simulink model "EHB_speedgoat_R2020a_V1"  (R2020a)
settings: Solver=FixedStepDiscrete  StartTime=0.0  StopTime=inf  FixedStep=0.001  RelTol=1e-3  EnableMultiTasking=on
model workspace (MAT data in the model file):
  A : Simulink.Signal (value not decoded)
  B : Simulink.Signal (value not decoded)
  C : Simulink.Signal (value not decoded)
  D : Simulink.Signal (value not decoded)
  E : Simulink.Signal (value not decoded)
  calin = [-9.96 -7.98 -5.98 -3.99 -1.994 0 1.995 3.992 5.99 7.98 9.97]
  calout = [-10 -8 -6 -4 -2 0 2 4 6 8 10]
symbols that are objects in the model workspace (value not decoded): C, D
undefined symbols (not defined in the file): Com1, none, ts_IO612
libraries: simulink x1436, xpcethercatlib x1223, yisutbxlib_utilities x256, xpcutilitieslib x156, hdlsllib x145, canmsglib x46, speedgoatlib_IO602_4 x11, speedgoatlib_IO611 x7, slrttcplib x4, CanManageLib x3, slrtlib x3, xpcseriallib x2
(part 4 of 30)

== system EHB_speedgoat_R2020a_V1/TIF_04/CB2020_2/mean11 ==
  In1 : Inport
  Add : Sum  Inputs=++++
  Add{1..4} (4 alike) : Sum  Inputs=++++++++++++++++++++
  Delay{,1..79} (80 alike) : Delay  DelayLength=1
  Gain : Gain  Gain=1/80
  Vol : Outport
  wires:
  Add/1 -> Gain/1
  Gain/1 -> Vol/1
  Delay36/1 -> Delay37/1, Add2/7
  Delay37/1 -> Delay38/1, Add2/8
  Delay34/1 -> Delay35/1, Add2/5
  Delay33/1 -> Delay34/1, Add2/4
  Delay20/1 -> Delay21/1, Add2/1
  Delay32/1 -> Delay33/1, Add2/3
  Add2/1 -> Add/2
  Delay35/1 -> Delay36/1, Add2/6
  Delay21/1 -> Delay32/1, Add2/2
  Delay38/1 -> Delay39/1, Add2/9
  Delay39/1 -> Delay22/1, Add2/10
  Delay19/1 -> Add1/20, Delay20/1
  Delay30/1 -> Delay31/1, Add2/19
  Delay23/1 -> Delay24/1, Add2/12
  Delay27/1 -> Delay28/1, Add2/16
  Delay24/1 -> Delay25/1, Add2/13
  Delay22/1 -> Delay23/1, Add2/11
  Delay25/1 -> Delay26/1, Add2/14
  Delay26/1 -> Delay27/1, Add2/15
  Delay29/1 -> Delay30/1, Add2/18
  Delay28/1 -> Delay29/1, Add2/17
  Delay16/1 -> Add1/17, Delay17/1
  Delay17/1 -> Add1/18, Delay18/1
  Delay14/1 -> Add1/15, Delay15/1
  Delay13/1 -> Add1/14, Delay14/1
  Delay10/1 -> Add1/11, Delay11/1
  Delay12/1 -> Add1/13, Delay13/1
  Delay15/1 -> Add1/16, Delay16/1
  Delay11/1 -> Add1/12, Delay12/1
  Delay18/1 -> Add1/19, Delay19/1
  In1/1 -> Delay/1
  Delay9/1 -> Add1/10, Delay10/1
  Delay8/1 -> Add1/9, Delay9/1
  Delay1/1 -> Add1/2, Delay2/1
  Delay5/1 -> Add1/6, Delay6/1
  Add1/1 -> Add/1
  Delay2/1 -> Add1/3, Delay3/1
  Delay/1 -> Add1/1, Delay1/1
  Delay3/1 -> Add1/4, Delay4/1
  Delay4/1 -> Add1/5, Delay5/1
  Delay7/1 -> Add1/8, Delay8/1
  Delay6/1 -> Add1/7, Delay7/1
  Delay48/1 -> Add3/17, Delay49/1
  Delay49/1 -> Add3/18, Delay50/1
  Delay46/1 -> Add3/15, Delay47/1
  Delay45/1 -> Add3/14, Delay46/1
  Delay42/1 -> Add3/11, Delay43/1
  Delay44/1 -> Add3/13, Delay45/1
  Delay47/1 -> Add3/16, Delay48/1
  Delay43/1 -> Add3/12, Delay44/1
  Delay50/1 -> Add3/19, Delay51/1
  Delay31/1 -> Delay40/1, Add2/20
  Delay59/1 -> Add3/10, Delay42/1
  Delay58/1 -> Add3/9, Delay59/1
  Delay41/1 -> Add3/2, Delay52/1
  Delay55/1 -> Add3/6, Delay56/1
  Add3/1 -> Add/3
  Delay52/1 -> Add3/3, Delay53/1
  Delay40/1 -> Add3/1, Delay41/1
  Delay53/1 -> Add3/4, Delay54/1
  Delay54/1 -> Add3/5, Delay55/1
  Delay57/1 -> Add3/8, Delay58/1
  Delay56/1 -> Add3/7, Delay57/1
  Delay76/1 -> Delay77/1, Add4/7
  Delay77/1 -> Delay78/1, Add4/8
  Delay74/1 -> Delay75/1, Add4/5
  Delay73/1 -> Delay74/1, Add4/4
  Delay60/1 -> Delay61/1, Add4/1
  Delay72/1 -> Delay73/1, Add4/3
  Add4/1 -> Add/4
  Delay75/1 -> Delay76/1, Add4/6
  Delay61/1 -> Delay72/1, Add4/2
  Delay78/1 -> Delay79/1, Add4/9
  Delay79/1 -> Delay62/1, Add4/10
  Delay71/1 -> Add4/20
  Delay51/1 -> Delay60/1, Add3/20
  Delay70/1 -> Delay71/1, Add4/19
  Delay63/1 -> Delay64/1, Add4/12
  Delay67/1 -> Delay68/1, Add4/16
  Delay64/1 -> Delay65/1, Add4/13
  Delay62/1 -> Delay63/1, Add4/11
  Delay65/1 -> Delay66/1, Add4/14
  Delay66/1 -> Delay67/1, Add4/15
  Delay69/1 -> Delay70/1, Add4/18
  Delay68/1 -> Delay69/1, Add4/17

== system EHB_speedgoat_R2020a_V1/TIF_04/CB2020_2/mean12 ==
  In1 : Inport
  Add : Sum  Inputs=++++
  Add{1..4} (4 alike) : Sum  Inputs=++++++++++++++++++++
  Delay{,1..79} (80 alike) : Delay  DelayLength=1
  Gain : Gain  Gain=1/80
  Vol : Outport
  wires:
  Delay68/1 -> Add4/17, Delay69/1
  Delay69/1 -> Add4/18, Delay70/1
  Delay66/1 -> Add4/15, Delay67/1
  Delay65/1 -> Add4/14, Delay66/1
  Delay62/1 -> Add4/11, Delay63/1
  Delay64/1 -> Add4/13, Delay65/1
  Delay67/1 -> Add4/16, Delay68/1
  Delay63/1 -> Add4/12, Delay64/1
  Delay70/1 -> Add4/19, Delay71/1
  Delay51/1 -> Add3/20, Delay60/1
  Delay71/1 -> Add4/20
  Delay79/1 -> Add4/10, Delay62/1
  Delay78/1 -> Add4/9, Delay79/1
  Delay61/1 -> Add4/2, Delay72/1
  Delay75/1 -> Add4/6, Delay76/1
  Add4/1 -> Add/4
  Delay72/1 -> Add4/3, Delay73/1
  Delay60/1 -> Add4/1, Delay61/1
  Delay73/1 -> Add4/4, Delay74/1
  Delay74/1 -> Add4/5, Delay75/1
  Delay77/1 -> Add4/8, Delay78/1
  Delay76/1 -> Add4/7, Delay77/1
  Delay56/1 -> Delay57/1, Add3/7
  Delay57/1 -> Delay58/1, Add3/8
  Delay54/1 -> Delay55/1, Add3/5
  Delay53/1 -> Delay54/1, Add3/4
  Delay40/1 -> Delay41/1, Add3/1
  Delay52/1 -> Delay53/1, Add3/3
  Add3/1 -> Add/3
  Delay55/1 -> Delay56/1, Add3/6
  Delay41/1 -> Delay52/1, Add3/2
  Delay58/1 -> Delay59/1, Add3/9
  Delay59/1 -> Delay42/1, Add3/10
  Delay31/1 -> Add2/20, Delay40/1
  Delay50/1 -> Delay51/1, Add3/19
  Delay43/1 -> Delay44/1, Add3/12
  Delay47/1 -> Delay48/1, Add3/16
  Delay44/1 -> Delay45/1, Add3/13
  Delay42/1 -> Delay43/1, Add3/11
  Delay45/1 -> Delay46/1, Add3/14
  Delay46/1 -> Delay47/1, Add3/15
  Delay49/1 -> Delay50/1, Add3/18
  Delay48/1 -> Delay49/1, Add3/17
  Delay6/1 -> Delay7/1, Add1/7
  Delay7/1 -> Delay8/1, Add1/8
  Delay4/1 -> Delay5/1, Add1/5
  Delay3/1 -> Delay4/1, Add1/4
  Delay/1 -> Delay1/1, Add1/1
  Delay2/1 -> Delay3/1, Add1/3
  Add1/1 -> Add/1
  Delay5/1 -> Delay6/1, Add1/6
  Delay1/1 -> Delay2/1, Add1/2
  Delay8/1 -> Delay9/1, Add1/9
  Delay9/1 -> Delay10/1, Add1/10
  In1/1 -> Delay/1
  Delay18/1 -> Delay19/1, Add1/19
  Delay11/1 -> Delay12/1, Add1/12
  Delay15/1 -> Delay16/1, Add1/16
  Delay12/1 -> Delay13/1, Add1/13
  Delay10/1 -> Delay11/1, Add1/11
  Delay13/1 -> Delay14/1, Add1/14
  Delay14/1 -> Delay15/1, Add1/15
  Delay17/1 -> Delay18/1, Add1/18
  Delay16/1 -> Delay17/1, Add1/17
  Delay28/1 -> Add2/17, Delay29/1
  Delay29/1 -> Add2/18, Delay30/1
  Delay26/1 -> Add2/15, Delay27/1
  Delay25/1 -> Add2/14, Delay26/1
  Delay22/1 -> Add2/11, Delay23/1
  Delay24/1 -> Add2/13, Delay25/1
  Delay27/1 -> Add2/16, Delay28/1
  Delay23/1 -> Add2/12, Delay24/1
  Delay30/1 -> Add2/19, Delay31/1
  Delay19/1 -> Delay20/1, Add1/20
  Delay39/1 -> Add2/10, Delay22/1
  Delay38/1 -> Add2/9, Delay39/1
  Delay21/1 -> Add2/2, Delay32/1
  Delay35/1 -> Add2/6, Delay36/1
  Add2/1 -> Add/2
  Delay32/1 -> Add2/3, Delay33/1
  Delay20/1 -> Add2/1, Delay21/1
  Delay33/1 -> Add2/4, Delay34/1
  Delay34/1 -> Add2/5, Delay35/1
  Delay37/1 -> Add2/8, Delay38/1
  Delay36/1 -> Add2/7, Delay37/1
  Gain/1 -> Vol/1
  Add/1 -> Gain/1

== system EHB_speedgoat_R2020a_V1/TIF_04/CB2020_2/mean13 ==
  In1 : Inport
  Add : Sum  Inputs=++++
  Add{1..4} (4 alike) : Sum  Inputs=++++++++++++++++++++
  Delay{,1..79} (80 alike) : Delay  DelayLength=1
  Gain : Gain  Gain=1/80
  Vol : Outport
  wires:
  Add/1 -> Gain/1
  Gain/1 -> Vol/1
  Delay36/1 -> Delay37/1, Add2/7
  Delay37/1 -> Delay38/1, Add2/8
  Delay34/1 -> Delay35/1, Add2/5
  Delay33/1 -> Delay34/1, Add2/4
  Delay20/1 -> Delay21/1, Add2/1
  Delay32/1 -> Delay33/1, Add2/3
  Add2/1 -> Add/2
  Delay35/1 -> Delay36/1, Add2/6
  Delay21/1 -> Delay32/1, Add2/2
  Delay38/1 -> Delay39/1, Add2/9
  Delay39/1 -> Delay22/1, Add2/10
  Delay19/1 -> Add1/20, Delay20/1
  Delay30/1 -> Delay31/1, Add2/19
  Delay23/1 -> Delay24/1, Add2/12
  Delay27/1 -> Delay28/1, Add2/16
  Delay24/1 -> Delay25/1, Add2/13
  Delay22/1 -> Delay23/1, Add2/11
  Delay25/1 -> Delay26/1, Add2/14
  Delay26/1 -> Delay27/1, Add2/15
  Delay29/1 -> Delay30/1, Add2/18
  Delay28/1 -> Delay29/1, Add2/17
  Delay16/1 -> Add1/17, Delay17/1
  Delay17/1 -> Add1/18, Delay18/1
  Delay14/1 -> Add1/15, Delay15/1
  Delay13/1 -> Add1/14, Delay14/1
  Delay10/1 -> Add1/11, Delay11/1
  Delay12/1 -> Add1/13, Delay13/1
  Delay15/1 -> Add1/16, Delay16/1
  Delay11/1 -> Add1/12, Delay12/1
  Delay18/1 -> Add1/19, Delay19/1
  In1/1 -> Delay/1
  Delay9/1 -> Add1/10, Delay10/1
  Delay8/1 -> Add1/9, Delay9/1
  Delay1/1 -> Add1/2, Delay2/1
  Delay5/1 -> Add1/6, Delay6/1
  Add1/1 -> Add/1
  Delay2/1 -> Add1/3, Delay3/1
  Delay/1 -> Add1/1, Delay1/1
  Delay3/1 -> Add1/4, Delay4/1
  Delay4/1 -> Add1/5, Delay5/1
  Delay7/1 -> Add1/8, Delay8/1
  Delay6/1 -> Add1/7, Delay7/1
  Delay48/1 -> Add3/17, Delay49/1
  Delay49/1 -> Add3/18, Delay50/1
  Delay46/1 -> Add3/15, Delay47/1
  Delay45/1 -> Add3/14, Delay46/1
  Delay42/1 -> Add3/11, Delay43/1
  Delay44/1 -> Add3/13, Delay45/1
  Delay47/1 -> Add3/16, Delay48/1
  Delay43/1 -> Add3/12, Delay44/1
  Delay50/1 -> Add3/19, Delay51/1
  Delay31/1 -> Delay40/1, Add2/20
  Delay59/1 -> Add3/10, Delay42/1
  Delay58/1 -> Add3/9, Delay59/1
  Delay41/1 -> Add3/2, Delay52/1
  Delay55/1 -> Add3/6, Delay56/1
  Add3/1 -> Add/3
  Delay52/1 -> Add3/3, Delay53/1
  Delay40/1 -> Add3/1, Delay41/1
  Delay53/1 -> Add3/4, Delay54/1
  Delay54/1 -> Add3/5, Delay55/1
  Delay57/1 -> Add3/8, Delay58/1
  Delay56/1 -> Add3/7, Delay57/1
  Delay76/1 -> Delay77/1, Add4/7
  Delay77/1 -> Delay78/1, Add4/8
  Delay74/1 -> Delay75/1, Add4/5
  Delay73/1 -> Delay74/1, Add4/4
  Delay60/1 -> Delay61/1, Add4/1
  Delay72/1 -> Delay73/1, Add4/3
  Add4/1 -> Add/4
  Delay75/1 -> Delay76/1, Add4/6
  Delay61/1 -> Delay72/1, Add4/2
  Delay78/1 -> Delay79/1, Add4/9
  Delay79/1 -> Delay62/1, Add4/10
  Delay71/1 -> Add4/20
  Delay51/1 -> Delay60/1, Add3/20
  Delay70/1 -> Delay71/1, Add4/19
  Delay63/1 -> Delay64/1, Add4/12
  Delay67/1 -> Delay68/1, Add4/16
  Delay64/1 -> Delay65/1, Add4/13
  Delay62/1 -> Delay63/1, Add4/11
  Delay65/1 -> Delay66/1, Add4/14
  Delay66/1 -> Delay67/1, Add4/15
  Delay69/1 -> Delay70/1, Add4/18
  Delay68/1 -> Delay69/1, Add4/17

== system EHB_speedgoat_R2020a_V1/TIF_04/CB2020_2/mean14 ==
  In1 : Inport
  Add : Sum  Inputs=++++
  Add{1..4} (4 alike) : Sum  Inputs=++++++++++++++++++++
  Delay{,1..79} (80 alike) : Delay  DelayLength=1
  Gain : Gain  Gain=1/80
  Vol : Outport
  wires:
  Delay68/1 -> Add4/17, Delay69/1
  Delay69/1 -> Add4/18, Delay70/1
  Delay66/1 -> Add4/15, Delay67/1
  Delay65/1 -> Add4/14, Delay66/1
  Delay62/1 -> Add4/11, Delay63/1
  Delay64/1 -> Add4/13, Delay65/1
  Delay67/1 -> Add4/16, Delay68/1
  Delay63/1 -> Add4/12, Delay64/1
  Delay70/1 -> Add4/19, Delay71/1
  Delay51/1 -> Add3/20, Delay60/1
  Delay71/1 -> Add4/20
  Delay79/1 -> Add4/10, Delay62/1
  Delay78/1 -> Add4/9, Delay79/1
  Delay61/1 -> Add4/2, Delay72/1
  Delay75/1 -> Add4/6, Delay76/1
  Add4/1 -> Add/4
  Delay72/1 -> Add4/3, Delay73/1
  Delay60/1 -> Add4/1, Delay61/1
  Delay73/1 -> Add4/4, Delay74/1
  Delay74/1 -> Add4/5, Delay75/1
  Delay77/1 -> Add4/8, Delay78/1
  Delay76/1 -> Add4/7, Delay77/1
  Delay56/1 -> Delay57/1, Add3/7
  Delay57/1 -> Delay58/1, Add3/8
  Delay54/1 -> Delay55/1, Add3/5
  Delay53/1 -> Delay54/1, Add3/4
  Delay40/1 -> Delay41/1, Add3/1
  Delay52/1 -> Delay53/1, Add3/3
  Add3/1 -> Add/3
  Delay55/1 -> Delay56/1, Add3/6
  Delay41/1 -> Delay52/1, Add3/2
  Delay58/1 -> Delay59/1, Add3/9
  Delay59/1 -> Delay42/1, Add3/10
  Delay31/1 -> Add2/20, Delay40/1
  Delay50/1 -> Delay51/1, Add3/19
  Delay43/1 -> Delay44/1, Add3/12
  Delay47/1 -> Delay48/1, Add3/16
  Delay44/1 -> Delay45/1, Add3/13
  Delay42/1 -> Delay43/1, Add3/11
  Delay45/1 -> Delay46/1, Add3/14
  Delay46/1 -> Delay47/1, Add3/15
  Delay49/1 -> Delay50/1, Add3/18
  Delay48/1 -> Delay49/1, Add3/17
  Delay6/1 -> Delay7/1, Add1/7
  Delay7/1 -> Delay8/1, Add1/8
  Delay4/1 -> Delay5/1, Add1/5
  Delay3/1 -> Delay4/1, Add1/4
  Delay/1 -> Delay1/1, Add1/1
  Delay2/1 -> Delay3/1, Add1/3
  Add1/1 -> Add/1
  Delay5/1 -> Delay6/1, Add1/6
  Delay1/1 -> Delay2/1, Add1/2
  Delay8/1 -> Delay9/1, Add1/9
  Delay9/1 -> Delay10/1, Add1/10
  In1/1 -> Delay/1
  Delay18/1 -> Delay19/1, Add1/19
  Delay11/1 -> Delay12/1, Add1/12
  Delay15/1 -> Delay16/1, Add1/16
  Delay12/1 -> Delay13/1, Add1/13
  Delay10/1 -> Delay11/1, Add1/11
  Delay13/1 -> Delay14/1, Add1/14
  Delay14/1 -> Delay15/1, Add1/15
  Delay17/1 -> Delay18/1, Add1/18
  Delay16/1 -> Delay17/1, Add1/17
  Delay28/1 -> Add2/17, Delay29/1
  Delay29/1 -> Add2/18, Delay30/1
  Delay26/1 -> Add2/15, Delay27/1
  Delay25/1 -> Add2/14, Delay26/1
  Delay22/1 -> Add2/11, Delay23/1
  Delay24/1 -> Add2/13, Delay25/1
  Delay27/1 -> Add2/16, Delay28/1
  Delay23/1 -> Add2/12, Delay24/1
  Delay30/1 -> Add2/19, Delay31/1
  Delay19/1 -> Delay20/1, Add1/20
  Delay39/1 -> Add2/10, Delay22/1
  Delay38/1 -> Add2/9, Delay39/1
  Delay21/1 -> Add2/2, Delay32/1
  Delay35/1 -> Add2/6, Delay36/1
  Add2/1 -> Add/2
  Delay32/1 -> Add2/3, Delay33/1
  Delay20/1 -> Add2/1, Delay21/1
  Delay33/1 -> Add2/4, Delay34/1
  Delay34/1 -> Add2/5, Delay35/1
  Delay37/1 -> Add2/8, Delay38/1
  Delay36/1 -> Add2/7, Delay37/1
  Gain/1 -> Vol/1
  Add/1 -> Gain/1

== system EHB_speedgoat_R2020a_V1/TIF_04/CB2020_2/mean15 ==
  In1 : Inport
  Add : Sum  Inputs=++++
  Add{1..4} (4 alike) : Sum  Inputs=++++++++++++++++++++
  Delay{,1..79} (80 alike) : Delay  DelayLength=1
  Gain : Gain  Gain=1/80
  Vol : Outport
  wires:
  Add/1 -> Gain/1
  Gain/1 -> Vol/1
  Delay36/1 -> Delay37/1, Add2/7
  Delay37/1 -> Delay38/1, Add2/8
  Delay34/1 -> Delay35/1, Add2/5
  Delay33/1 -> Delay34/1, Add2/4
  Delay20/1 -> Delay21/1, Add2/1
  Delay32/1 -> Delay33/1, Add2/3
  Add2/1 -> Add/2
  Delay35/1 -> Delay36/1, Add2/6
  Delay21/1 -> Delay32/1, Add2/2
  Delay38/1 -> Delay39/1, Add2/9
  Delay39/1 -> Delay22/1, Add2/10
  Delay19/1 -> Add1/20, Delay20/1
  Delay30/1 -> Delay31/1, Add2/19
  Delay23/1 -> Delay24/1, Add2/12
  Delay27/1 -> Delay28/1, Add2/16
  Delay24/1 -> Delay25/1, Add2/13
  Delay22/1 -> Delay23/1, Add2/11
  Delay25/1 -> Delay26/1, Add2/14
  Delay26/1 -> Delay27/1, Add2/15
  Delay29/1 -> Delay30/1, Add2/18
  Delay28/1 -> Delay29/1, Add2/17
  Delay16/1 -> Add1/17, Delay17/1
  Delay17/1 -> Add1/18, Delay18/1
  Delay14/1 -> Add1/15, Delay15/1
  Delay13/1 -> Add1/14, Delay14/1
  Delay10/1 -> Add1/11, Delay11/1
  Delay12/1 -> Add1/13, Delay13/1
  Delay15/1 -> Add1/16, Delay16/1
  Delay11/1 -> Add1/12, Delay12/1
  Delay18/1 -> Add1/19, Delay19/1
  In1/1 -> Delay/1
  Delay9/1 -> Add1/10, Delay10/1
  Delay8/1 -> Add1/9, Delay9/1
  Delay1/1 -> Add1/2, Delay2/1
  Delay5/1 -> Add1/6, Delay6/1
  Add1/1 -> Add/1
  Delay2/1 -> Add1/3, Delay3/1
  Delay/1 -> Add1/1, Delay1/1
  Delay3/1 -> Add1/4, Delay4/1
  Delay4/1 -> Add1/5, Delay5/1
  Delay7/1 -> Add1/8, Delay8/1
  Delay6/1 -> Add1/7, Delay7/1
  Delay48/1 -> Add3/17, Delay49/1
  Delay49/1 -> Add3/18, Delay50/1
  Delay46/1 -> Add3/15, Delay47/1
  Delay45/1 -> Add3/14, Delay46/1
  Delay42/1 -> Add3/11, Delay43/1
  Delay44/1 -> Add3/13, Delay45/1
  Delay47/1 -> Add3/16, Delay48/1
  Delay43/1 -> Add3/12, Delay44/1
  Delay50/1 -> Add3/19, Delay51/1
  Delay31/1 -> Delay40/1, Add2/20
  Delay59/1 -> Add3/10, Delay42/1
  Delay58/1 -> Add3/9, Delay59/1
  Delay41/1 -> Add3/2, Delay52/1
  Delay55/1 -> Add3/6, Delay56/1
  Add3/1 -> Add/3
  Delay52/1 -> Add3/3, Delay53/1
  Delay40/1 -> Add3/1, Delay41/1
  Delay53/1 -> Add3/4, Delay54/1
  Delay54/1 -> Add3/5, Delay55/1
  Delay57/1 -> Add3/8, Delay58/1
  Delay56/1 -> Add3/7, Delay57/1
  Delay76/1 -> Delay77/1, Add4/7
  Delay77/1 -> Delay78/1, Add4/8
  Delay74/1 -> Delay75/1, Add4/5
  Delay73/1 -> Delay74/1, Add4/4
  Delay60/1 -> Delay61/1, Add4/1
  Delay72/1 -> Delay73/1, Add4/3
  Add4/1 -> Add/4
  Delay75/1 -> Delay76/1, Add4/6
  Delay61/1 -> Delay72/1, Add4/2
  Delay78/1 -> Delay79/1, Add4/9
  Delay79/1 -> Delay62/1, Add4/10
  Delay71/1 -> Add4/20
  Delay51/1 -> Delay60/1, Add3/20
  Delay70/1 -> Delay71/1, Add4/19
  Delay63/1 -> Delay64/1, Add4/12
  Delay67/1 -> Delay68/1, Add4/16
  Delay64/1 -> Delay65/1, Add4/13
  Delay62/1 -> Delay63/1, Add4/11
  Delay65/1 -> Delay66/1, Add4/14
  Delay66/1 -> Delay67/1, Add4/15
  Delay69/1 -> Delay70/1, Add4/18
  Delay68/1 -> Delay69/1, Add4/17

== system EHB_speedgoat_R2020a_V1/TIF_04/CB2020_2/mean16 ==
  In1 : Inport
  Add : Sum  Inputs=++++
  Add{1..4} (4 alike) : Sum  Inputs=++++++++++++++++++++
  Delay{,1..79} (80 alike) : Delay  DelayLength=1
  Gain : Gain  Gain=1/80
  Vol : Outport
  wires:
  Delay68/1 -> Add4/17, Delay69/1
  Delay69/1 -> Add4/18, Delay70/1
  Delay66/1 -> Add4/15, Delay67/1
  Delay65/1 -> Add4/14, Delay66/1
  Delay62/1 -> Add4/11, Delay63/1
  Delay64/1 -> Add4/13, Delay65/1
  Delay67/1 -> Add4/16, Delay68/1
  Delay63/1 -> Add4/12, Delay64/1
  Delay70/1 -> Add4/19, Delay71/1
  Delay51/1 -> Add3/20, Delay60/1
  Delay71/1 -> Add4/20
  Delay79/1 -> Add4/10, Delay62/1
  Delay78/1 -> Add4/9, Delay79/1
  Delay61/1 -> Add4/2, Delay72/1
  Delay75/1 -> Add4/6, Delay76/1
  Add4/1 -> Add/4
  Delay72/1 -> Add4/3, Delay73/1
  Delay60/1 -> Add4/1, Delay61/1
  Delay73/1 -> Add4/4, Delay74/1
  Delay74/1 -> Add4/5, Delay75/1
  Delay77/1 -> Add4/8, Delay78/1
  Delay76/1 -> Add4/7, Delay77/1
  Delay56/1 -> Delay57/1, Add3/7
  Delay57/1 -> Delay58/1, Add3/8
  Delay54/1 -> Delay55/1, Add3/5
  Delay53/1 -> Delay54/1, Add3/4
  Delay40/1 -> Delay41/1, Add3/1
  Delay52/1 -> Delay53/1, Add3/3
  Add3/1 -> Add/3
  Delay55/1 -> Delay56/1, Add3/6
  Delay41/1 -> Delay52/1, Add3/2
  Delay58/1 -> Delay59/1, Add3/9
  Delay59/1 -> Delay42/1, Add3/10
  Delay31/1 -> Add2/20, Delay40/1
  Delay50/1 -> Delay51/1, Add3/19
  Delay43/1 -> Delay44/1, Add3/12
  Delay47/1 -> Delay48/1, Add3/16
  Delay44/1 -> Delay45/1, Add3/13
  Delay42/1 -> Delay43/1, Add3/11
  Delay45/1 -> Delay46/1, Add3/14
  Delay46/1 -> Delay47/1, Add3/15
  Delay49/1 -> Delay50/1, Add3/18
  Delay48/1 -> Delay49/1, Add3/17
  Delay6/1 -> Delay7/1, Add1/7
  Delay7/1 -> Delay8/1, Add1/8
  Delay4/1 -> Delay5/1, Add1/5
  Delay3/1 -> Delay4/1, Add1/4
  Delay/1 -> Delay1/1, Add1/1
  Delay2/1 -> Delay3/1, Add1/3
  Add1/1 -> Add/1
  Delay5/1 -> Delay6/1, Add1/6
  Delay1/1 -> Delay2/1, Add1/2
  Delay8/1 -> Delay9/1, Add1/9
  Delay9/1 -> Delay10/1, Add1/10
  In1/1 -> Delay/1
  Delay18/1 -> Delay19/1, Add1/19
  Delay11/1 -> Delay12/1, Add1/12
  Delay15/1 -> Delay16/1, Add1/16
  Delay12/1 -> Delay13/1, Add1/13
  Delay10/1 -> Delay11/1, Add1/11
  Delay13/1 -> Delay14/1, Add1/14
  Delay14/1 -> Delay15/1, Add1/15
  Delay17/1 -> Delay18/1, Add1/18
  Delay16/1 -> Delay17/1, Add1/17
  Delay28/1 -> Add2/17, Delay29/1
  Delay29/1 -> Add2/18, Delay30/1
  Delay26/1 -> Add2/15, Delay27/1
  Delay25/1 -> Add2/14, Delay26/1
  Delay22/1 -> Add2/11, Delay23/1
  Delay24/1 -> Add2/13, Delay25/1
  Delay27/1 -> Add2/16, Delay28/1
  Delay23/1 -> Add2/12, Delay24/1
  Delay30/1 -> Add2/19, Delay31/1
  Delay19/1 -> Delay20/1, Add1/20
  Delay39/1 -> Add2/10, Delay22/1
  Delay38/1 -> Add2/9, Delay39/1
  Delay21/1 -> Add2/2, Delay32/1
  Delay35/1 -> Add2/6, Delay36/1
  Add2/1 -> Add/2
  Delay32/1 -> Add2/3, Delay33/1
  Delay20/1 -> Add2/1, Delay21/1
  Delay33/1 -> Add2/4, Delay34/1
  Delay34/1 -> Add2/5, Delay35/1
  Delay37/1 -> Add2/8, Delay38/1
  Delay36/1 -> Add2/7, Delay37/1
  Gain/1 -> Vol/1
  Add/1 -> Gain/1

== system EHB_speedgoat_R2020a_V1/TIF_04/CB2020_2/mean2 ==
  In1 : Inport
  Add : Sum  Inputs=++++
  Add{1..4} (4 alike) : Sum  Inputs=++++++++++++++++++++
  Delay{,1..79} (80 alike) : Delay  DelayLength=1
  Gain : Gain  Gain=1/80
  Vol : Outport
  wires:
  Delay68/1 -> Add4/17, Delay69/1
  Delay69/1 -> Add4/18, Delay70/1
  Delay66/1 -> Add4/15, Delay67/1
  Delay65/1 -> Add4/14, Delay66/1
  Delay62/1 -> Add4/11, Delay63/1
  Delay64/1 -> Add4/13, Delay65/1
  Delay67/1 -> Add4/16, Delay68/1
  Delay63/1 -> Add4/12, Delay64/1
  Delay70/1 -> Add4/19, Delay71/1
  Delay51/1 -> Add3/20, Delay60/1
  Delay71/1 -> Add4/20
  Delay79/1 -> Add4/10, Delay62/1
  Delay78/1 -> Add4/9, Delay79/1
  Delay61/1 -> Add4/2, Delay72/1
  Delay75/1 -> Add4/6, Delay76/1
  Add4/1 -> Add/4
  Delay72/1 -> Add4/3, Delay73/1
  Delay60/1 -> Add4/1, Delay61/1
  Delay73/1 -> Add4/4, Delay74/1
  Delay74/1 -> Add4/5, Delay75/1
  Delay77/1 -> Add4/8, Delay78/1
  Delay76/1 -> Add4/7, Delay77/1
  Delay56/1 -> Delay57/1, Add3/7
  Delay57/1 -> Delay58/1, Add3/8
  Delay54/1 -> Delay55/1, Add3/5
  Delay53/1 -> Delay54/1, Add3/4
  Delay40/1 -> Delay41/1, Add3/1
  Delay52/1 -> Delay53/1, Add3/3
  Add3/1 -> Add/3
  Delay55/1 -> Delay56/1, Add3/6
  Delay41/1 -> Delay52/1, Add3/2
  Delay58/1 -> Delay59/1, Add3/9
  Delay59/1 -> Delay42/1, Add3/10
  Delay31/1 -> Add2/20, Delay40/1
  Delay50/1 -> Delay51/1, Add3/19
  Delay43/1 -> Delay44/1, Add3/12
  Delay47/1 -> Delay48/1, Add3/16
  Delay44/1 -> Delay45/1, Add3/13
  Delay42/1 -> Delay43/1, Add3/11
  Delay45/1 -> Delay46/1, Add3/14
  Delay46/1 -> Delay47/1, Add3/15
  Delay49/1 -> Delay50/1, Add3/18
  Delay48/1 -> Delay49/1, Add3/17
  Delay6/1 -> Delay7/1, Add1/7
  Delay7/1 -> Delay8/1, Add1/8
  Delay4/1 -> Delay5/1, Add1/5
  Delay3/1 -> Delay4/1, Add1/4
  Delay/1 -> Delay1/1, Add1/1
  Delay2/1 -> Delay3/1, Add1/3
  Add1/1 -> Add/1
  Delay5/1 -> Delay6/1, Add1/6
  Delay1/1 -> Delay2/1, Add1/2
  Delay8/1 -> Delay9/1, Add1/9
  Delay9/1 -> Delay10/1, Add1/10
  In1/1 -> Delay/1
  Delay18/1 -> Delay19/1, Add1/19
  Delay11/1 -> Delay12/1, Add1/12
  Delay15/1 -> Delay16/1, Add1/16
  Delay12/1 -> Delay13/1, Add1/13
  Delay10/1 -> Delay11/1, Add1/11
  Delay13/1 -> Delay14/1, Add1/14
  Delay14/1 -> Delay15/1, Add1/15
  Delay17/1 -> Delay18/1, Add1/18
  Delay16/1 -> Delay17/1, Add1/17
  Delay28/1 -> Add2/17, Delay29/1
  Delay29/1 -> Add2/18, Delay30/1
  Delay26/1 -> Add2/15, Delay27/1
  Delay25/1 -> Add2/14, Delay26/1
  Delay22/1 -> Add2/11, Delay23/1
  Delay24/1 -> Add2/13, Delay25/1
  Delay27/1 -> Add2/16, Delay28/1
  Delay23/1 -> Add2/12, Delay24/1
  Delay30/1 -> Add2/19, Delay31/1
  Delay19/1 -> Delay20/1, Add1/20
  Delay39/1 -> Add2/10, Delay22/1
  Delay38/1 -> Add2/9, Delay39/1
  Delay21/1 -> Add2/2, Delay32/1
  Delay35/1 -> Add2/6, Delay36/1
  Add2/1 -> Add/2
  Delay32/1 -> Add2/3, Delay33/1
  Delay20/1 -> Add2/1, Delay21/1
  Delay33/1 -> Add2/4, Delay34/1
  Delay34/1 -> Add2/5, Delay35/1
  Delay37/1 -> Add2/8, Delay38/1
  Delay36/1 -> Add2/7, Delay37/1
  Gain/1 -> Vol/1
  Add/1 -> Gain/1

== system EHB_speedgoat_R2020a_V1/TIF_04/CB2020_2/mean3 ==
  In1 : Inport
  Add : Sum  Inputs=++++
  Add{1..4} (4 alike) : Sum  Inputs=++++++++++++++++++++
  Delay{,1..79} (80 alike) : Delay  DelayLength=1
  Gain : Gain  Gain=1/80
  Vol : Outport
  wires:
  Add/1 -> Gain/1
  Gain/1 -> Vol/1
  Delay36/1 -> Delay37/1, Add2/7
  Delay37/1 -> Delay38/1, Add2/8
  Delay34/1 -> Delay35/1, Add2/5
  Delay33/1 -> Delay34/1, Add2/4
  Delay20/1 -> Delay21/1, Add2/1
  Delay32/1 -> Delay33/1, Add2/3
  Add2/1 -> Add/2
  Delay35/1 -> Delay36/1, Add2/6
  Delay21/1 -> Delay32/1, Add2/2
  Delay38/1 -> Delay39/1, Add2/9
  Delay39/1 -> Delay22/1, Add2/10
  Delay19/1 -> Add1/20, Delay20/1
  Delay30/1 -> Delay31/1, Add2/19
  Delay23/1 -> Delay24/1, Add2/12
  Delay27/1 -> Delay28/1, Add2/16
  Delay24/1 -> Delay25/1, Add2/13
  Delay22/1 -> Delay23/1, Add2/11
  Delay25/1 -> Delay26/1, Add2/14
  Delay26/1 -> Delay27/1, Add2/15
  Delay29/1 -> Delay30/1, Add2/18
  Delay28/1 -> Delay29/1, Add2/17
  Delay16/1 -> Add1/17, Delay17/1
  Delay17/1 -> Add1/18, Delay18/1
  Delay14/1 -> Add1/15, Delay15/1
  Delay13/1 -> Add1/14, Delay14/1
  Delay10/1 -> Add1/11, Delay11/1
  Delay12/1 -> Add1/13, Delay13/1
  Delay15/1 -> Add1/16, Delay16/1
  Delay11/1 -> Add1/12, Delay12/1
  Delay18/1 -> Add1/19, Delay19/1
  In1/1 -> Delay/1
  Delay9/1 -> Add1/10, Delay10/1
  Delay8/1 -> Add1/9, Delay9/1
  Delay1/1 -> Add1/2, Delay2/1
  Delay5/1 -> Add1/6, Delay6/1
  Add1/1 -> Add/1
  Delay2/1 -> Add1/3, Delay3/1
  Delay/1 -> Add1/1, Delay1/1
  Delay3/1 -> Add1/4, Delay4/1
  Delay4/1 -> Add1/5, Delay5/1
  Delay7/1 -> Add1/8, Delay8/1
  Delay6/1 -> Add1/7, Delay7/1
  Delay48/1 -> Add3/17, Delay49/1
  Delay49/1 -> Add3/18, Delay50/1
  Delay46/1 -> Add3/15, Delay47/1
  Delay45/1 -> Add3/14, Delay46/1
  Delay42/1 -> Add3/11, Delay43/1
  Delay44/1 -> Add3/13, Delay45/1
  Delay47/1 -> Add3/16, Delay48/1
  Delay43/1 -> Add3/12, Delay44/1
  Delay50/1 -> Add3/19, Delay51/1
  Delay31/1 -> Delay40/1, Add2/20
  Delay59/1 -> Add3/10, Delay42/1
  Delay58/1 -> Add3/9, Delay59/1
  Delay41/1 -> Add3/2, Delay52/1
  Delay55/1 -> Add3/6, Delay56/1
  Add3/1 -> Add/3
  Delay52/1 -> Add3/3, Delay53/1
  Delay40/1 -> Add3/1, Delay41/1
  Delay53/1 -> Add3/4, Delay54/1
  Delay54/1 -> Add3/5, Delay55/1
  Delay57/1 -> Add3/8, Delay58/1
  Delay56/1 -> Add3/7, Delay57/1
  Delay76/1 -> Delay77/1, Add4/7
  Delay77/1 -> Delay78/1, Add4/8
  Delay74/1 -> Delay75/1, Add4/5
  Delay73/1 -> Delay74/1, Add4/4
  Delay60/1 -> Delay61/1, Add4/1
  Delay72/1 -> Delay73/1, Add4/3
  Add4/1 -> Add/4
  Delay75/1 -> Delay76/1, Add4/6
  Delay61/1 -> Delay72/1, Add4/2
  Delay78/1 -> Delay79/1, Add4/9
  Delay79/1 -> Delay62/1, Add4/10
  Delay71/1 -> Add4/20
  Delay51/1 -> Delay60/1, Add3/20
  Delay70/1 -> Delay71/1, Add4/19
  Delay63/1 -> Delay64/1, Add4/12
  Delay67/1 -> Delay68/1, Add4/16
  Delay64/1 -> Delay65/1, Add4/13
  Delay62/1 -> Delay63/1, Add4/11
  Delay65/1 -> Delay66/1, Add4/14
  Delay66/1 -> Delay67/1, Add4/15
  Delay69/1 -> Delay70/1, Add4/18
  Delay68/1 -> Delay69/1, Add4/17

== system EHB_speedgoat_R2020a_V1/TIF_04/CB2020_2/mean4 ==
  In1 : Inport
  Add : Sum  Inputs=++++
  Add{1..4} (4 alike) : Sum  Inputs=++++++++++++++++++++
  Delay{,1..79} (80 alike) : Delay  DelayLength=1
  Gain : Gain  Gain=1/80
  Vol : Outport
  wires:
  Delay68/1 -> Add4/17, Delay69/1
  Delay69/1 -> Add4/18, Delay70/1
  Delay66/1 -> Add4/15, Delay67/1
  Delay65/1 -> Add4/14, Delay66/1
  Delay62/1 -> Add4/11, Delay63/1
  Delay64/1 -> Add4/13, Delay65/1
  Delay67/1 -> Add4/16, Delay68/1
  Delay63/1 -> Add4/12, Delay64/1
  Delay70/1 -> Add4/19, Delay71/1
  Delay51/1 -> Add3/20, Delay60/1
  Delay71/1 -> Add4/20
  Delay79/1 -> Add4/10, Delay62/1
  Delay78/1 -> Add4/9, Delay79/1
  Delay61/1 -> Add4/2, Delay72/1
  Delay75/1 -> Add4/6, Delay76/1
  Add4/1 -> Add/4
  Delay72/1 -> Add4/3, Delay73/1
  Delay60/1 -> Add4/1, Delay61/1
  Delay73/1 -> Add4/4, Delay74/1
  Delay74/1 -> Add4/5, Delay75/1
  Delay77/1 -> Add4/8, Delay78/1
  Delay76/1 -> Add4/7, Delay77/1
  Delay56/1 -> Delay57/1, Add3/7
  Delay57/1 -> Delay58/1, Add3/8
  Delay54/1 -> Delay55/1, Add3/5
  Delay53/1 -> Delay54/1, Add3/4
  Delay40/1 -> Delay41/1, Add3/1
  Delay52/1 -> Delay53/1, Add3/3
  Add3/1 -> Add/3
  Delay55/1 -> Delay56/1, Add3/6
  Delay41/1 -> Delay52/1, Add3/2
  Delay58/1 -> Delay59/1, Add3/9
  Delay59/1 -> Delay42/1, Add3/10
  Delay31/1 -> Add2/20, Delay40/1
  Delay50/1 -> Delay51/1, Add3/19
  Delay43/1 -> Delay44/1, Add3/12
  Delay47/1 -> Delay48/1, Add3/16
  Delay44/1 -> Delay45/1, Add3/13
  Delay42/1 -> Delay43/1, Add3/11
  Delay45/1 -> Delay46/1, Add3/14
  Delay46/1 -> Delay47/1, Add3/15
  Delay49/1 -> Delay50/1, Add3/18
  Delay48/1 -> Delay49/1, Add3/17
  Delay6/1 -> Delay7/1, Add1/7
  Delay7/1 -> Delay8/1, Add1/8
  Delay4/1 -> Delay5/1, Add1/5
  Delay3/1 -> Delay4/1, Add1/4
  Delay/1 -> Delay1/1, Add1/1
  Delay2/1 -> Delay3/1, Add1/3
  Add1/1 -> Add/1
  Delay5/1 -> Delay6/1, Add1/6
  Delay1/1 -> Delay2/1, Add1/2
  Delay8/1 -> Delay9/1, Add1/9
  Delay9/1 -> Delay10/1, Add1/10
  In1/1 -> Delay/1
  Delay18/1 -> Delay19/1, Add1/19
  Delay11/1 -> Delay12/1, Add1/12
  Delay15/1 -> Delay16/1, Add1/16
  Delay12/1 -> Delay13/1, Add1/13
  Delay10/1 -> Delay11/1, Add1/11
  Delay13/1 -> Delay14/1, Add1/14
  Delay14/1 -> Delay15/1, Add1/15
  Delay17/1 -> Delay18/1, Add1/18
  Delay16/1 -> Delay17/1, Add1/17
  Delay28/1 -> Add2/17, Delay29/1
  Delay29/1 -> Add2/18, Delay30/1
  Delay26/1 -> Add2/15, Delay27/1
  Delay25/1 -> Add2/14, Delay26/1
  Delay22/1 -> Add2/11, Delay23/1
  Delay24/1 -> Add2/13, Delay25/1
  Delay27/1 -> Add2/16, Delay28/1
  Delay23/1 -> Add2/12, Delay24/1
  Delay30/1 -> Add2/19, Delay31/1
  Delay19/1 -> Delay20/1, Add1/20
  Delay39/1 -> Add2/10, Delay22/1
  Delay38/1 -> Add2/9, Delay39/1
  Delay21/1 -> Add2/2, Delay32/1
  Delay35/1 -> Add2/6, Delay36/1
  Add2/1 -> Add/2
  Delay32/1 -> Add2/3, Delay33/1
  Delay20/1 -> Add2/1, Delay21/1
  Delay33/1 -> Add2/4, Delay34/1
  Delay34/1 -> Add2/5, Delay35/1
  Delay37/1 -> Add2/8, Delay38/1
  Delay36/1 -> Add2/7, Delay37/1
  Gain/1 -> Vol/1
  Add/1 -> Gain/1

== system EHB_speedgoat_R2020a_V1/TIF_04/CB2020_2/mean5 ==
  In1 : Inport
  Add : Sum  Inputs=++++
  Add{1..4} (4 alike) : Sum  Inputs=++++++++++++++++++++
  Delay{,1..79} (80 alike) : Delay  DelayLength=1
  Gain : Gain  Gain=1/80
  Vol : Outport
  wires:
  Add/1 -> Gain/1
  Gain/1 -> Vol/1
  Delay36/1 -> Delay37/1, Add2/7
  Delay37/1 -> Delay38/1, Add2/8
  Delay34/1 -> Delay35/1, Add2/5
  Delay33/1 -> Delay34/1, Add2/4
  Delay20/1 -> Delay21/1, Add2/1
  Delay32/1 -> Delay33/1, Add2/3
  Add2/1 -> Add/2
  Delay35/1 -> Delay36/1, Add2/6
  Delay21/1 -> Delay32/1, Add2/2
  Delay38/1 -> Delay39/1, Add2/9
  Delay39/1 -> Delay22/1, Add2/10
  Delay19/1 -> Add1/20, Delay20/1
  Delay30/1 -> Delay31/1, Add2/19
  Delay23/1 -> Delay24/1, Add2/12
  Delay27/1 -> Delay28/1, Add2/16
  Delay24/1 -> Delay25/1, Add2/13
  Delay22/1 -> Delay23/1, Add2/11
  Delay25/1 -> Delay26/1, Add2/14
  Delay26/1 -> Delay27/1, Add2/15
  Delay29/1 -> Delay30/1, Add2/18
  Delay28/1 -> Delay29/1, Add2/17
  Delay16/1 -> Add1/17, Delay17/1
  Delay17/1 -> Add1/18, Delay18/1
  Delay14/1 -> Add1/15, Delay15/1
  Delay13/1 -> Add1/14, Delay14/1
  Delay10/1 -> Add1/11, Delay11/1
  Delay12/1 -> Add1/13, Delay13/1
  Delay15/1 -> Add1/16, Delay16/1
  Delay11/1 -> Add1/12, Delay12/1
  Delay18/1 -> Add1/19, Delay19/1
  In1/1 -> Delay/1
  Delay9/1 -> Add1/10, Delay10/1
  Delay8/1 -> Add1/9, Delay9/1
  Delay1/1 -> Add1/2, Delay2/1
  Delay5/1 -> Add1/6, Delay6/1
  Add1/1 -> Add/1
  Delay2/1 -> Add1/3, Delay3/1
  Delay/1 -> Add1/1, Delay1/1
  Delay3/1 -> Add1/4, Delay4/1
  Delay4/1 -> Add1/5, Delay5/1
  Delay7/1 -> Add1/8, Delay8/1
  Delay6/1 -> Add1/7, Delay7/1
  Delay48/1 -> Add3/17, Delay49/1
  Delay49/1 -> Add3/18, Delay50/1
  Delay46/1 -> Add3/15, Delay47/1
  Delay45/1 -> Add3/14, Delay46/1
  Delay42/1 -> Add3/11, Delay43/1
  Delay44/1 -> Add3/13, Delay45/1
  Delay47/1 -> Add3/16, Delay48/1
  Delay43/1 -> Add3/12, Delay44/1
  Delay50/1 -> Add3/19, Delay51/1
  Delay31/1 -> Delay40/1, Add2/20
  Delay59/1 -> Add3/10, Delay42/1
  Delay58/1 -> Add3/9, Delay59/1
  Delay41/1 -> Add3/2, Delay52/1
  Delay55/1 -> Add3/6, Delay56/1
  Add3/1 -> Add/3
  Delay52/1 -> Add3/3, Delay53/1
  Delay40/1 -> Add3/1, Delay41/1
  Delay53/1 -> Add3/4, Delay54/1
  Delay54/1 -> Add3/5, Delay55/1
  Delay57/1 -> Add3/8, Delay58/1
  Delay56/1 -> Add3/7, Delay57/1
  Delay76/1 -> Delay77/1, Add4/7
  Delay77/1 -> Delay78/1, Add4/8
  Delay74/1 -> Delay75/1, Add4/5
  Delay73/1 -> Delay74/1, Add4/4
  Delay60/1 -> Delay61/1, Add4/1
  Delay72/1 -> Delay73/1, Add4/3
  Add4/1 -> Add/4
  Delay75/1 -> Delay76/1, Add4/6
  Delay61/1 -> Delay72/1, Add4/2
  Delay78/1 -> Delay79/1, Add4/9
  Delay79/1 -> Delay62/1, Add4/10
  Delay71/1 -> Add4/20
  Delay51/1 -> Delay60/1, Add3/20
  Delay70/1 -> Delay71/1, Add4/19
  Delay63/1 -> Delay64/1, Add4/12
  Delay67/1 -> Delay68/1, Add4/16
  Delay64/1 -> Delay65/1, Add4/13
  Delay62/1 -> Delay63/1, Add4/11
  Delay65/1 -> Delay66/1, Add4/14
  Delay66/1 -> Delay67/1, Add4/15
  Delay69/1 -> Delay70/1, Add4/18
  Delay68/1 -> Delay69/1, Add4/17

== system EHB_speedgoat_R2020a_V1/TIF_04/CB2020_2/mean6 ==
  In1 : Inport
  Add : Sum  Inputs=++++
  Add{1..4} (4 alike) : Sum  Inputs=++++++++++++++++++++
  Delay{,1..79} (80 alike) : Delay  DelayLength=1
  Gain : Gain  Gain=1/80
  Vol : Outport
  wires:
  Delay68/1 -> Add4/17, Delay69/1
  Delay69/1 -> Add4/18, Delay70/1
  Delay66/1 -> Add4/15, Delay67/1
  Delay65/1 -> Add4/14, Delay66/1
  Delay62/1 -> Add4/11, Delay63/1
  Delay64/1 -> Add4/13, Delay65/1
  Delay67/1 -> Add4/16, Delay68/1
  Delay63/1 -> Add4/12, Delay64/1
  Delay70/1 -> Add4/19, Delay71/1
  Delay51/1 -> Add3/20, Delay60/1
  Delay71/1 -> Add4/20
  Delay79/1 -> Add4/10, Delay62/1
  Delay78/1 -> Add4/9, Delay79/1
  Delay61/1 -> Add4/2, Delay72/1
  Delay75/1 -> Add4/6, Delay76/1
  Add4/1 -> Add/4
  Delay72/1 -> Add4/3, Delay73/1
  Delay60/1 -> Add4/1, Delay61/1
  Delay73/1 -> Add4/4, Delay74/1
  Delay74/1 -> Add4/5, Delay75/1
  Delay77/1 -> Add4/8, Delay78/1
  Delay76/1 -> Add4/7, Delay77/1
  Delay56/1 -> Delay57/1, Add3/7
  Delay57/1 -> Delay58/1, Add3/8
  Delay54/1 -> Delay55/1, Add3/5
  Delay53/1 -> Delay54/1, Add3/4
  Delay40/1 -> Delay41/1, Add3/1
  Delay52/1 -> Delay53/1, Add3/3
  Add3/1 -> Add/3
  Delay55/1 -> Delay56/1, Add3/6
  Delay41/1 -> Delay52/1, Add3/2
  Delay58/1 -> Delay59/1, Add3/9
  Delay59/1 -> Delay42/1, Add3/10
  Delay31/1 -> Add2/20, Delay40/1
  Delay50/1 -> Delay51/1, Add3/19
  Delay43/1 -> Delay44/1, Add3/12
  Delay47/1 -> Delay48/1, Add3/16
  Delay44/1 -> Delay45/1, Add3/13
  Delay42/1 -> Delay43/1, Add3/11
  Delay45/1 -> Delay46/1, Add3/14
  Delay46/1 -> Delay47/1, Add3/15
  Delay49/1 -> Delay50/1, Add3/18
  Delay48/1 -> Delay49/1, Add3/17
  Delay6/1 -> Delay7/1, Add1/7
  Delay7/1 -> Delay8/1, Add1/8
  Delay4/1 -> Delay5/1, Add1/5
  Delay3/1 -> Delay4/1, Add1/4
  Delay/1 -> Delay1/1, Add1/1
  Delay2/1 -> Delay3/1, Add1/3
  Add1/1 -> Add/1
  Delay5/1 -> Delay6/1, Add1/6
  Delay1/1 -> Delay2/1, Add1/2
  Delay8/1 -> Delay9/1, Add1/9
  Delay9/1 -> Delay10/1, Add1/10
  In1/1 -> Delay/1
  Delay18/1 -> Delay19/1, Add1/19
  Delay11/1 -> Delay12/1, Add1/12
  Delay15/1 -> Delay16/1, Add1/16
  Delay12/1 -> Delay13/1, Add1/13
  Delay10/1 -> Delay11/1, Add1/11
  Delay13/1 -> Delay14/1, Add1/14
  Delay14/1 -> Delay15/1, Add1/15
  Delay17/1 -> Delay18/1, Add1/18
  Delay16/1 -> Delay17/1, Add1/17
  Delay28/1 -> Add2/17, Delay29/1
  Delay29/1 -> Add2/18, Delay30/1
  Delay26/1 -> Add2/15, Delay27/1
  Delay25/1 -> Add2/14, Delay26/1
  Delay22/1 -> Add2/11, Delay23/1
  Delay24/1 -> Add2/13, Delay25/1
  Delay27/1 -> Add2/16, Delay28/1
  Delay23/1 -> Add2/12, Delay24/1
  Delay30/1 -> Add2/19, Delay31/1
  Delay19/1 -> Delay20/1, Add1/20
  Delay39/1 -> Add2/10, Delay22/1
  Delay38/1 -> Add2/9, Delay39/1
  Delay21/1 -> Add2/2, Delay32/1
  Delay35/1 -> Add2/6, Delay36/1
  Add2/1 -> Add/2
  Delay32/1 -> Add2/3, Delay33/1
  Delay20/1 -> Add2/1, Delay21/1
  Delay33/1 -> Add2/4, Delay34/1
  Delay34/1 -> Add2/5, Delay35/1
  Delay37/1 -> Add2/8, Delay38/1
  Delay36/1 -> Add2/7, Delay37/1
  Gain/1 -> Vol/1
  Add/1 -> Gain/1

== system EHB_speedgoat_R2020a_V1/TIF_04/CB2020_2/mean7 ==
  In1 : Inport
  Add : Sum  Inputs=++++
  Add{1..4} (4 alike) : Sum  Inputs=++++++++++++++++++++
  Delay{,1..79} (80 alike) : Delay  DelayLength=1
  Gain : Gain  Gain=1/80
  Vol : Outport
  wires:
  Add/1 -> Gain/1
  Gain/1 -> Vol/1
  Delay36/1 -> Delay37/1, Add2/7
  Delay37/1 -> Delay38/1, Add2/8
  Delay34/1 -> Delay35/1, Add2/5
  Delay33/1 -> Delay34/1, Add2/4
  Delay20/1 -> Delay21/1, Add2/1
  Delay32/1 -> Delay33/1, Add2/3
  Add2/1 -> Add/2
  Delay35/1 -> Delay36/1, Add2/6
  Delay21/1 -> Delay32/1, Add2/2
  Delay38/1 -> Delay39/1, Add2/9
  Delay39/1 -> Delay22/1, Add2/10
  Delay19/1 -> Add1/20, Delay20/1
  Delay30/1 -> Delay31/1, Add2/19
  Delay23/1 -> Delay24/1, Add2/12
  Delay27/1 -> Delay28/1, Add2/16
  Delay24/1 -> Delay25/1, Add2/13
  Delay22/1 -> Delay23/1, Add2/11
  Delay25/1 -> Delay26/1, Add2/14
  Delay26/1 -> Delay27/1, Add2/15
  Delay29/1 -> Delay30/1, Add2/18
  Delay28/1 -> Delay29/1, Add2/17
  Delay16/1 -> Add1/17, Delay17/1
  Delay17/1 -> Add1/18, Delay18/1
  Delay14/1 -> Add1/15, Delay15/1
  Delay13/1 -> Add1/14, Delay14/1
  Delay10/1 -> Add1/11, Delay11/1
  Delay12/1 -> Add1/13, Delay13/1
  Delay15/1 -> Add1/16, Delay16/1
  Delay11/1 -> Add1/12, Delay12/1
  Delay18/1 -> Add1/19, Delay19/1
  In1/1 -> Delay/1
  Delay9/1 -> Add1/10, Delay10/1
  Delay8/1 -> Add1/9, Delay9/1
  Delay1/1 -> Add1/2, Delay2/1
  Delay5/1 -> Add1/6, Delay6/1
  Add1/1 -> Add/1
  Delay2/1 -> Add1/3, Delay3/1
  Delay/1 -> Add1/1, Delay1/1
  Delay3/1 -> Add1/4, Delay4/1
  Delay4/1 -> Add1/5, Delay5/1
  Delay7/1 -> Add1/8, Delay8/1
  Delay6/1 -> Add1/7, Delay7/1
  Delay48/1 -> Add3/17, Delay49/1
  Delay49/1 -> Add3/18, Delay50/1
  Delay46/1 -> Add3/15, Delay47/1
  Delay45/1 -> Add3/14, Delay46/1
  Delay42/1 -> Add3/11, Delay43/1
  Delay44/1 -> Add3/13, Delay45/1
  Delay47/1 -> Add3/16, Delay48/1
  Delay43/1 -> Add3/12, Delay44/1
  Delay50/1 -> Add3/19, Delay51/1
  Delay31/1 -> Delay40/1, Add2/20
  Delay59/1 -> Add3/10, Delay42/1
  Delay58/1 -> Add3/9, Delay59/1
  Delay41/1 -> Add3/2, Delay52/1
  Delay55/1 -> Add3/6, Delay56/1
  Add3/1 -> Add/3
  Delay52/1 -> Add3/3, Delay53/1
  Delay40/1 -> Add3/1, Delay41/1
  Delay53/1 -> Add3/4, Delay54/1
  Delay54/1 -> Add3/5, Delay55/1
  Delay57/1 -> Add3/8, Delay58/1
  Delay56/1 -> Add3/7, Delay57/1
  Delay76/1 -> Delay77/1, Add4/7
  Delay77/1 -> Delay78/1, Add4/8
  Delay74/1 -> Delay75/1, Add4/5
  Delay73/1 -> Delay74/1, Add4/4
  Delay60/1 -> Delay61/1, Add4/1
  Delay72/1 -> Delay73/1, Add4/3
  Add4/1 -> Add/4
  Delay75/1 -> Delay76/1, Add4/6
  Delay61/1 -> Delay72/1, Add4/2
  Delay78/1 -> Delay79/1, Add4/9
  Delay79/1 -> Delay62/1, Add4/10
  Delay71/1 -> Add4/20
  Delay51/1 -> Delay60/1, Add3/20
  Delay70/1 -> Delay71/1, Add4/19
  Delay63/1 -> Delay64/1, Add4/12
  Delay67/1 -> Delay68/1, Add4/16
  Delay64/1 -> Delay65/1, Add4/13
  Delay62/1 -> Delay63/1, Add4/11
  Delay65/1 -> Delay66/1, Add4/14
  Delay66/1 -> Delay67/1, Add4/15
  Delay69/1 -> Delay70/1, Add4/18
  Delay68/1 -> Delay69/1, Add4/17

== system EHB_speedgoat_R2020a_V1/TIF_04/CB2020_2/mean8 ==
  In1 : Inport
  Add : Sum  Inputs=++++
  Add{1..4} (4 alike) : Sum  Inputs=++++++++++++++++++++
  Delay{,1..79} (80 alike) : Delay  DelayLength=1
  Gain : Gain  Gain=1/80
  Vol : Outport
  wires:
  Delay68/1 -> Add4/17, Delay69/1
  Delay69/1 -> Add4/18, Delay70/1
  Delay66/1 -> Add4/15, Delay67/1
  Delay65/1 -> Add4/14, Delay66/1
  Delay62/1 -> Add4/11, Delay63/1
  Delay64/1 -> Add4/13, Delay65/1
  Delay67/1 -> Add4/16, Delay68/1
  Delay63/1 -> Add4/12, Delay64/1
  Delay70/1 -> Add4/19, Delay71/1
  Delay51/1 -> Add3/20, Delay60/1
  Delay71/1 -> Add4/20
  Delay79/1 -> Add4/10, Delay62/1
  Delay78/1 -> Add4/9, Delay79/1
  Delay61/1 -> Add4/2, Delay72/1
  Delay75/1 -> Add4/6, Delay76/1
  Add4/1 -> Add/4
  Delay72/1 -> Add4/3, Delay73/1
  Delay60/1 -> Add4/1, Delay61/1
  Delay73/1 -> Add4/4, Delay74/1
  Delay74/1 -> Add4/5, Delay75/1
  Delay77/1 -> Add4/8, Delay78/1
  Delay76/1 -> Add4/7, Delay77/1
  Delay56/1 -> Delay57/1, Add3/7
  Delay57/1 -> Delay58/1, Add3/8
  Delay54/1 -> Delay55/1, Add3/5
  Delay53/1 -> Delay54/1, Add3/4
  Delay40/1 -> Delay41/1, Add3/1
  Delay52/1 -> Delay53/1, Add3/3
  Add3/1 -> Add/3
  Delay55/1 -> Delay56/1, Add3/6
  Delay41/1 -> Delay52/1, Add3/2
  Delay58/1 -> Delay59/1, Add3/9
  Delay59/1 -> Delay42/1, Add3/10
  Delay31/1 -> Add2/20, Delay40/1
  Delay50/1 -> Delay51/1, Add3/19
  Delay43/1 -> Delay44/1, Add3/12
  Delay47/1 -> Delay48/1, Add3/16
  Delay44/1 -> Delay45/1, Add3/13
  Delay42/1 -> Delay43/1, Add3/11
  Delay45/1 -> Delay46/1, Add3/14
  Delay46/1 -> Delay47/1, Add3/15
  Delay49/1 -> Delay50/1, Add3/18
  Delay48/1 -> Delay49/1, Add3/17
  Delay6/1 -> Delay7/1, Add1/7
  Delay7/1 -> Delay8/1, Add1/8
  Delay4/1 -> Delay5/1, Add1/5
  Delay3/1 -> Delay4/1, Add1/4
  Delay/1 -> Delay1/1, Add1/1
  Delay2/1 -> Delay3/1, Add1/3
  Add1/1 -> Add/1
  Delay5/1 -> Delay6/1, Add1/6
  Delay1/1 -> Delay2/1, Add1/2
  Delay8/1 -> Delay9/1, Add1/9
  Delay9/1 -> Delay10/1, Add1/10
  In1/1 -> Delay/1
  Delay18/1 -> Delay19/1, Add1/19
  Delay11/1 -> Delay12/1, Add1/12
  Delay15/1 -> Delay16/1, Add1/16
  Delay12/1 -> Delay13/1, Add1/13
  Delay10/1 -> Delay11/1, Add1/11
  Delay13/1 -> Delay14/1, Add1/14
  Delay14/1 -> Delay15/1, Add1/15
  Delay17/1 -> Delay18/1, Add1/18
  Delay16/1 -> Delay17/1, Add1/17
  Delay28/1 -> Add2/17, Delay29/1
  Delay29/1 -> Add2/18, Delay30/1
  Delay26/1 -> Add2/15, Delay27/1
  Delay25/1 -> Add2/14, Delay26/1
  Delay22/1 -> Add2/11, Delay23/1
  Delay24/1 -> Add2/13, Delay25/1
  Delay27/1 -> Add2/16, Delay28/1
  Delay23/1 -> Add2/12, Delay24/1
  Delay30/1 -> Add2/19, Delay31/1
  Delay19/1 -> Delay20/1, Add1/20
  Delay39/1 -> Add2/10, Delay22/1
  Delay38/1 -> Add2/9, Delay39/1
  Delay21/1 -> Add2/2, Delay32/1
  Delay35/1 -> Add2/6, Delay36/1
  Add2/1 -> Add/2
  Delay32/1 -> Add2/3, Delay33/1
  Delay20/1 -> Add2/1, Delay21/1
  Delay33/1 -> Add2/4, Delay34/1
  Delay34/1 -> Add2/5, Delay35/1
  Delay37/1 -> Add2/8, Delay38/1
  Delay36/1 -> Add2/7, Delay37/1
  Gain/1 -> Vol/1
  Add/1 -> Gain/1

== system EHB_speedgoat_R2020a_V1/TIF_04/CB2020_2/mean9 ==
  In1 : Inport
  Add : Sum  Inputs=++++
  Add{1..4} (4 alike) : Sum  Inputs=++++++++++++++++++++
  Delay{,1..79} (80 alike) : Delay  DelayLength=1
  Gain : Gain  Gain=1/80
  Vol : Outport
  wires:
  Add/1 -> Gain/1
  Gain/1 -> Vol/1
  Delay36/1 -> Delay37/1, Add2/7
  Delay37/1 -> Delay38/1, Add2/8
  Delay34/1 -> Delay35/1, Add2/5
  Delay33/1 -> Delay34/1, Add2/4
  Delay20/1 -> Delay21/1, Add2/1
  Delay32/1 -> Delay33/1, Add2/3
  Add2/1 -> Add/2
  Delay35/1 -> Delay36/1, Add2/6
  Delay21/1 -> Delay32/1, Add2/2
  Delay38/1 -> Delay39/1, Add2/9
  Delay39/1 -> Delay22/1, Add2/10
  Delay19/1 -> Add1/20, Delay20/1
  Delay30/1 -> Delay31/1, Add2/19
  Delay23/1 -> Delay24/1, Add2/12
  Delay27/1 -> Delay28/1, Add2/16
  Delay24/1 -> Delay25/1, Add2/13
  Delay22/1 -> Delay23/1, Add2/11
  Delay25/1 -> Delay26/1, Add2/14
  Delay26/1 -> Delay27/1, Add2/15
  Delay29/1 -> Delay30/1, Add2/18
  Delay28/1 -> Delay29/1, Add2/17
  Delay16/1 -> Add1/17, Delay17/1
  Delay17/1 -> Add1/18, Delay18/1
  Delay14/1 -> Add1/15, Delay15/1
  Delay13/1 -> Add1/14, Delay14/1
  Delay10/1 -> Add1/11, Delay11/1
  Delay12/1 -> Add1/13, Delay13/1
  Delay15/1 -> Add1/16, Delay16/1
  Delay11/1 -> Add1/12, Delay12/1
  Delay18/1 -> Add1/19, Delay19/1
  In1/1 -> Delay/1
  Delay9/1 -> Add1/10, Delay10/1
  Delay8/1 -> Add1/9, Delay9/1
  Delay1/1 -> Add1/2, Delay2/1
  Delay5/1 -> Add1/6, Delay6/1
  Add1/1 -> Add/1
  Delay2/1 -> Add1/3, Delay3/1
  Delay/1 -> Add1/1, Delay1/1
  Delay3/1 -> Add1/4, Delay4/1
  Delay4/1 -> Add1/5, Delay5/1
  Delay7/1 -> Add1/8, Delay8/1
  Delay6/1 -> Add1/7, Delay7/1
  Delay48/1 -> Add3/17, Delay49/1
  Delay49/1 -> Add3/18, Delay50/1
  Delay46/1 -> Add3/15, Delay47/1
  Delay45/1 -> Add3/14, Delay46/1
  Delay42/1 -> Add3/11, Delay43/1
  Delay44/1 -> Add3/13, Delay45/1
  Delay47/1 -> Add3/16, Delay48/1
  Delay43/1 -> Add3/12, Delay44/1
  Delay50/1 -> Add3/19, Delay51/1
  Delay31/1 -> Delay40/1, Add2/20
  Delay59/1 -> Add3/10, Delay42/1
  Delay58/1 -> Add3/9, Delay59/1
  Delay41/1 -> Add3/2, Delay52/1
  Delay55/1 -> Add3/6, Delay56/1
  Add3/1 -> Add/3
  Delay52/1 -> Add3/3, Delay53/1
  Delay40/1 -> Add3/1, Delay41/1
  Delay53/1 -> Add3/4, Delay54/1
  Delay54/1 -> Add3/5, Delay55/1
  Delay57/1 -> Add3/8, Delay58/1
  Delay56/1 -> Add3/7, Delay57/1
  Delay76/1 -> Delay77/1, Add4/7
  Delay77/1 -> Delay78/1, Add4/8
  Delay74/1 -> Delay75/1, Add4/5
  Delay73/1 -> Delay74/1, Add4/4
  Delay60/1 -> Delay61/1, Add4/1
  Delay72/1 -> Delay73/1, Add4/3
  Add4/1 -> Add/4
  Delay75/1 -> Delay76/1, Add4/6
  Delay61/1 -> Delay72/1, Add4/2
  Delay78/1 -> Delay79/1, Add4/9
  Delay79/1 -> Delay62/1, Add4/10
  Delay71/1 -> Add4/20
  Delay51/1 -> Delay60/1, Add3/20
  Delay70/1 -> Delay71/1, Add4/19
  Delay63/1 -> Delay64/1, Add4/12
  Delay67/1 -> Delay68/1, Add4/16
  Delay64/1 -> Delay65/1, Add4/13
  Delay62/1 -> Delay63/1, Add4/11
  Delay65/1 -> Delay66/1, Add4/14
  Delay66/1 -> Delay67/1, Add4/15
  Delay69/1 -> Delay70/1, Add4/18
  Delay68/1 -> Delay69/1, Add4/17

== system EHB_speedgoat_R2020a_V1/TIF_04/CB2020_3/ADC ==
  DTCB CH5 : DataTypeConversion  OutDataTypeStr=double
  EtherCAT PDO Receive ADC CH5 : xpcethercatlib/EtherCAT PDO Receive  Priority=2  sig_name=Box 7 (CB2020).PDOGetValue process data mapping.adcvalue5  sig_offset=11512  sig_type=uint16  type_size=16  sig_dim=1  device_id=0  sample_time=0.001000
      settings: SourceProductBaseCode=XP
  Gain CH5 : Gain  Gain=1/1000
  ADC_CH5[V] : Outport
  wires:
  EtherCAT PDO Receive ADC CH5/1 -> DTCB CH5/1
  DTCB CH5/1 -> Gain CH5/1
  Gain CH5/1 -> ADC_CH5[V]/1  "ADC_CH5[V]"

== system EHB_speedgoat_R2020a_V1/TIF_04/CB2020_3/AI1 ==
  Vol : Inport
  Add : Sum  Inputs=-+
  Constant : Constant  Value=5.002
  V2A : Gain  Gain=1/0.1  OutDataTypeStr=Inherit: Inherit via back propagation
  Cur : Outport
  wires:
  Add/1 -> V2A/1
  Vol/1 -> Add/2
  Constant/1 -> Add/1
  V2A/1 -> Cur/1

== system EHB_speedgoat_R2020a_V1/TIF_04/CB2020_3/AI2 ==
  Vol : Inport
  Add : Sum  Inputs=-+
  Constant : Constant  Value=4.9953
  V2A : Gain  Gain=1/0.1  OutDataTypeStr=Inherit: Inherit via back propagation
  Cur : Outport
  wires:
  V2A/1 -> Cur/1
  Constant/1 -> Add/1
  Vol/1 -> Add/2
  Add/1 -> V2A/1

== system EHB_speedgoat_R2020a_V1/TIF_04/CB2020_3/AI3 ==
  Vol : Inport
  Add : Sum  Inputs=-+
  Constant : Constant  Value=5.0068
  V2A : Gain  Gain=1/0.1  OutDataTypeStr=Inherit: Inherit via back propagation
  Cur : Outport
  wires:
  Add/1 -> V2A/1
  Vol/1 -> Add/2
  Constant/1 -> Add/1
  V2A/1 -> Cur/1

== system EHB_speedgoat_R2020a_V1/TIF_04/CB2020_3/AI4 ==
  Vol : Inport
  Add : Sum  Inputs=-+
  Constant : Constant  Value=5.0152
  V2A : Gain  Gain=1/0.1  OutDataTypeStr=Inherit: Inherit via back propagation
  Cur : Outport
  wires:
  V2A/1 -> Cur/1
  Constant/1 -> Add/1
  Vol/1 -> Add/2
  Add/1 -> V2A/1

== system EHB_speedgoat_R2020a_V1/TIF_04/CB2020_3/DAC1 ==
  DAC_CH1[V] : Inport
  DAC_CH1_CAL[V] : Constant  Value=0
  EtherCAT PDO Transmit DAC CH1 : xpcethercatlib/EtherCAT PDO Transmit   Priority=3  sig_name=Box 7 (CB2020).PDOSetValue process data mapping.dacvalue1  sig_offset=11448  sig_type=int16  type_size=16  sig_dim=1  device_id=0  sample_time=0.001000
      settings: SourceProductBaseCode=XP
  dp2c CH1 : Subsystem  mask(dacphy2cmd){}
  wires:
  DAC_CH1[V]/1 -> dp2c CH1/1(dac_value)
  DAC_CH1_CAL[V]/1 -> dp2c CH1/2(dac_value_calibrate)
  dp2c CH1/1(cmd_value) -> EtherCAT PDO Transmit DAC CH1/1

== system EHB_speedgoat_R2020a_V1/TIF_04/CB2020_3/Sw ==
  In2 : Inport
  In3 : Inport  Port=2
  Vol : Inport  Port=3
  Add : Sum
  Add1 : Sum
  Constant : Constant  Value=0.02
  Constant1 : Constant  Value=0.01
  Switch : Switch  Criteria=u2 > Threshold  Threshold=2.2
  Out1 : Outport
  wires:
  Constant/1 -> Add/2
  Add/1 -> Switch/3
  Add1/1 -> Switch/1
  Switch/1 -> Out1/1
  In3/1 -> Add/1
  In2/1 -> Switch/2
  Constant1/1 -> Add1/1
  Vol/1 -> Add1/2

== system EHB_speedgoat_R2020a_V1/TIF_04/CB2020_3/Sw1 ==
  In2 : Inport
  In3 : Inport  Port=2
  Vol : Inport  Port=3
  Add : Sum
  Add1 : Sum
  Constant : Constant  Value=0.02
  Constant1 : Constant  Value=0.01
  Switch : Switch  Criteria=u2 > Threshold  Threshold=2.2
  Out1 : Outport
  wires:
  In2/1 -> Switch/2
  In3/1 -> Add/1
  Switch/1 -> Out1/1
  Add1/1 -> Switch/1
  Add/1 -> Switch/3
  Constant/1 -> Add/2
  Constant1/1 -> Add1/1
  Vol/1 -> Add1/2

== system EHB_speedgoat_R2020a_V1/TIF_04/CB2020_3/Sw10 ==
  In2 : Inport
  In3 : Inport  Port=2
  Vol : Inport  Port=3
  Add : Sum
  Add1 : Sum
  Constant : Constant  Value=0.02
  Constant1 : Constant  Value=0.01
  Switch : Switch  Criteria=u2 > Threshold  Threshold=2.2
  Out1 : Outport
  wires:
  In2/1 -> Switch/2
  In3/1 -> Add/1
  Switch/1 -> Out1/1
  Add1/1 -> Switch/1
  Add/1 -> Switch/3
  Constant/1 -> Add/2
  Constant1/1 -> Add1/1
  Vol/1 -> Add1/2

== system EHB_speedgoat_R2020a_V1/TIF_04/CB2020_3/Sw11 ==
  In2 : Inport
  In3 : Inport  Port=2
  Vol : Inport  Port=3
  Add : Sum
  Add1 : Sum
  Constant : Constant  Value=0.02
  Constant1 : Constant  Value=0.01
  Switch : Switch  Criteria=u2 > Threshold  Threshold=2.2
  Out1 : Outport
  wires:
  Constant/1 -> Add/2
  Add/1 -> Switch/3
  Add1/1 -> Switch/1
  Switch/1 -> Out1/1
  In3/1 -> Add/1
  In2/1 -> Switch/2
  Constant1/1 -> Add1/1
  Vol/1 -> Add1/2

== system EHB_speedgoat_R2020a_V1/TIF_04/CB2020_3/Sw2 ==
  In2 : Inport
  In3 : Inport  Port=2
  Vol : Inport  Port=3
  Add : Sum
  Add1 : Sum
  Constant : Constant  Value=0.015
  Constant1 : Constant  Value=0.01
  Switch : Switch  Criteria=u2 > Threshold  Threshold=2.2
  Out1 : Outport
  wires:
  Constant/1 -> Add/2
  Add/1 -> Switch/3
  Add1/1 -> Switch/1
  Switch/1 -> Out1/1
  In3/1 -> Add/1
  In2/1 -> Switch/2
  Constant1/1 -> Add1/1
  Vol/1 -> Add1/2

== system EHB_speedgoat_R2020a_V1/TIF_04/CB2020_3/Sw3 ==
  In2 : Inport
  In3 : Inport  Port=2
  Vol : Inport  Port=3
  Add : Sum
  Add1 : Sum
  Constant : Constant  Value=0.02
  Constant1 : Constant  Value=0.01
  Switch : Switch  Criteria=u2 > Threshold  Threshold=2.2
  Out1 : Outport
  wires:
  In2/1 -> Switch/2
  In3/1 -> Add/1
  Switch/1 -> Out1/1
  Add1/1 -> Switch/1
  Add/1 -> Switch/3
  Constant/1 -> Add/2
  Constant1/1 -> Add1/1
  Vol/1 -> Add1/2

== system EHB_speedgoat_R2020a_V1/TIF_04/CB2020_3/Sw4 ==
  In2 : Inport
  In3 : Inport  Port=2
  Vol : Inport  Port=3
  Add : Sum
  Add1 : Sum
  Constant : Constant  Value=0.02
  Constant1 : Constant  Value=0.01
  Switch : Switch  Criteria=u2 > Threshold  Threshold=2.2
  Out1 : Outport
  wires:
  Constant/1 -> Add/2
  Add/1 -> Switch/3
  Add1/1 -> Switch/1
  Switch/1 -> Out1/1
  In3/1 -> Add/1
  In2/1 -> Switch/2
  Constant1/1 -> Add1/1
  Vol/1 -> Add1/2

== system EHB_speedgoat_R2020a_V1/TIF_04/CB2020_3/Sw5 ==
  In2 : Inport
  In3 : Inport  Port=2
  Vol : Inport  Port=3
  Add : Sum
  Add1 : Sum
  Constant : Constant  Value=0.02
  Constant1 : Constant  Value=0.01
  Switch : Switch  Criteria=u2 > Threshold  Threshold=2.2
  Out1 : Outport
  wires:
  Switch/1 -> Out1/1
  Add1/1 -> Switch/1
  Add/1 -> Switch/3
  Constant/1 -> Add/2
  Constant1/1 -> Add1/1
  In2/1 -> Add1/2
  In3/1 -> Switch/2
  Vol/1 -> Add/1
